simulink model "msfun_test"  (R2017b)
settings: Solver=VariableStepAuto  StartTime=0.0  StopTime=10.0  RelTol=1e-3
settings Model: Creator=Michele  LastModifiedBy=Michele

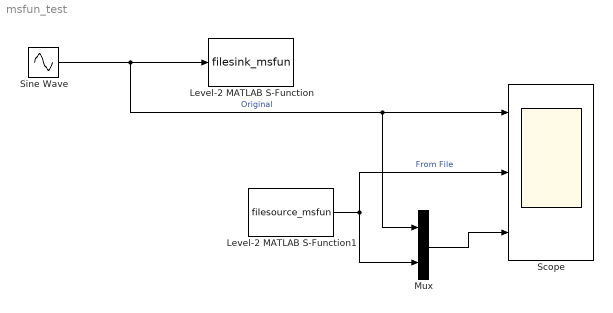
== system msfun_test ==
  Level-2 MATLAB S-Function : M-S-Function  FunctionName=filesink_msfun
  Level-2 MATLAB S-Function1 : M-S-Function  FunctionName=filesource_msfun
  Mux : Mux  Inputs=2
  Scope : Scope  NumInputPorts=3
  Sine Wave : Sin  SampleTime=0
  wires:
  Sine Wave/1 -> Mux/1, Scope/1, Level-2 MATLAB S-Function/1  "Original"
  Level-2 MATLAB S-Function1/1 -> Scope/2, Mux/2  "From File"
  Mux/1 -> Scope/3
